simulink library "halout"  (R2021b)
settings: Solver=VariableStepAuto  StartTime=0.0  StopTime=10.0  RelTol=1e-3
undefined symbols (not defined in the file): C_TASK_5MS_S, FALSE, KHAL_CAN1TxReq_flg, KHAL_CAN2TxReq_flg, KHAL_CAN3FD3VCU1toNIDECTxReq_flg, KHAL_CAN3FD3VCU1TxReq_flg, KHAL_CAN3FD3VCU2E2E_flg, KHAL_CAN3FD3VCU2toNIDECE2E_flg, KHAL_CAN3FD3VCU2toNIDECTxReq_flg, KHAL_CAN3FD3VCU2TxReq_flg, KHAL_CAN3TxReq_flg, KHAL_CAN4FD4CE1000E2E_flg, KHAL_CAN4FD4CE1000TxReq_flg, KHAL_CAN4TxReq_flg, KHAL_CAN5TxReq_flg, KHAL_CAN7TxReq_flg, ONE_INT, TRUE, ZERO_INT
libraries: FVT_lib x258, simulink x115
(part 12 of 17)

== system halout/HAL_OUT/CAN3/FD3_THCM1_0x182/BatteryMode ==
  BatteryMode : Inport
  Data Type Conversion : DataTypeConversion  OutDataTypeStr=uint8  RndMeth=Round
  CAN3_BatteryMode : Outport
  wires:
  Data Type Conversion/1 -> CAN3_BatteryMode/1
  BatteryMode/1 -> Data Type Conversion/1

== system halout/HAL_OUT/CAN3/FD3_THCM1_0x182/CCUACLampSts ==
  CCUACLampSts : Inport
  Data Type Conversion : DataTypeConversion  OutDataTypeStr=uint8  RndMeth=Round
  CAN3_CCU_ACLampSts : Outport
  wires:
  Data Type Conversion/1 -> CAN3_CCU_ACLampSts/1
  CCUACLampSts/1 -> Data Type Conversion/1

== system halout/HAL_OUT/CAN3/FD3_THCM1_0x182/CCUACMaxLampSts ==
  CCUACMaxLampSts : Inport
  Data Type Conversion : DataTypeConversion  OutDataTypeStr=uint8  RndMeth=Round
  CAN3_CCU_ACMaxLampSts : Outport
  wires:
  Data Type Conversion/1 -> CAN3_CCU_ACMaxLampSts/1
  CCUACMaxLampSts/1 -> Data Type Conversion/1

== system halout/HAL_OUT/CAN3/FD3_THCM1_0x182/CCUAutoLampSts ==
  CCUAutoLampSts : Inport
  Data Type Conversion : DataTypeConversion  OutDataTypeStr=uint8  RndMeth=Round
  CAN3_CCU_AutoLampSts : Outport
  wires:
  Data Type Conversion/1 -> CAN3_CCU_AutoLampSts/1
  CCUAutoLampSts/1 -> Data Type Conversion/1

== system halout/HAL_OUT/CAN3/FD3_THCM1_0x182/CCUAutoMidLampSts ==
  CCUAutoMidLampSts : Inport
  Data Type Conversion : DataTypeConversion  OutDataTypeStr=uint8  RndMeth=Round
  CAN3_CCU_AutoMidLampSts : Outport
  wires:
  Data Type Conversion/1 -> CAN3_CCU_AutoMidLampSts/1
  CCUAutoMidLampSts/1 -> Data Type Conversion/1

== system halout/HAL_OUT/CAN3/FD3_THCM1_0x182/CCUDispalyRequest ==
  CCUDispalyRequest : Inport
  Data Type Conversion : DataTypeConversion  OutDataTypeStr=uint8  RndMeth=Round
  CAN3_CCU_Dispaly_Request : Outport
  wires:
  Data Type Conversion/1 -> CAN3_CCU_Dispaly_Request/1
  CCUDispalyRequest/1 -> Data Type Conversion/1

== system halout/HAL_OUT/CAN3/FD3_THCM1_0x182/CCUEcoSts ==
  CCUEcoSts : Inport
  Data Type Conversion : DataTypeConversion  OutDataTypeStr=uint8  RndMeth=Round
  CAN3_CCU_EcoSts : Outport
  wires:
  Data Type Conversion/1 -> CAN3_CCU_EcoSts/1
  CCUEcoSts/1 -> Data Type Conversion/1

== system halout/HAL_OUT/CAN3/FD3_THCM1_0x182/CCUFrtOnOffLampSts ==
  CCUFrtOnOffLampSts : Inport
  Data Type Conversion : DataTypeConversion  OutDataTypeStr=uint8  RndMeth=Round
  CAN3_CCU_FrtOnOffLampSts : Outport
  wires:
  Data Type Conversion/1 -> CAN3_CCU_FrtOnOffLampSts/1
  CCUFrtOnOffLampSts/1 -> Data Type Conversion/1

== system halout/HAL_OUT/CAN3/FD3_THCM1_0x182/CCUHEATMaxLampSts ==
  CCUHEATMaxLampSts : Inport
  Data Type Conversion : DataTypeConversion  OutDataTypeStr=uint8  RndMeth=Round
  CAN3_CCU_HEATMaxLampSts : Outport
  wires:
  Data Type Conversion/1 -> CAN3_CCU_HEATMaxLampSts/1
  CCUHEATMaxLampSts/1 -> Data Type Conversion/1

== system halout/HAL_OUT/CAN3/FD3_THCM1_0x182/CCURrOnOffLampSts ==
  CCURrOnOffLampSts : Inport
  Data Type Conversion : DataTypeConversion  OutDataTypeStr=uint8  RndMeth=Round
  CAN3_CCU_RrOnOffLampSts : Outport
  wires:
  Data Type Conversion/1 -> CAN3_CCU_RrOnOffLampSts/1
  CCURrOnOffLampSts/1 -> Data Type Conversion/1

== system halout/HAL_OUT/CAN3/FD3_THCM1_0x182/CCUSyncLampSts ==
  CCUSyncLampSts : Inport
  Data Type Conversion : DataTypeConversion  OutDataTypeStr=uint8  RndMeth=Round
  CAN3_CCU_SyncLampSts : Outport
  wires:
  Data Type Conversion/1 -> CAN3_CCU_SyncLampSts/1
  CCUSyncLampSts/1 -> Data Type Conversion/1

== system halout/HAL_OUT/CAN3/FD3_THCM1_0x182/CabinMode ==
  CabinMode : Inport
  Data Type Conversion : DataTypeConversion  OutDataTypeStr=uint8  RndMeth=Round
  CAN3_CabinMode : Outport
  wires:
  Data Type Conversion/1 -> CAN3_CabinMode/1
  CabinMode/1 -> Data Type Conversion/1

== system halout/HAL_OUT/CAN3/FD3_THCM1_0x182/EDriveMode ==
  EDriveMode : Inport
  Data Type Conversion : DataTypeConversion  OutDataTypeStr=uint8  RndMeth=Round
  CAN3_EDriveMode : Outport
  wires:
  Data Type Conversion/1 -> CAN3_EDriveMode/1
  EDriveMode/1 -> Data Type Conversion/1

== system halout/HAL_OUT/CAN3/FD3_THCM1_0x182/FDAGSCmd ==
  FDAGSCmd : Inport
  Data Type Conversion : DataTypeConversion  OutDataTypeStr=uint8  RndMeth=Round
  CAN3_FD_AGS_Cmd : Outport
  wires:
  Data Type Conversion/1 -> CAN3_FD_AGS_Cmd/1
  FDAGSCmd/1 -> Data Type Conversion/1

== system halout/HAL_OUT/CAN3/FD3_THCM1_0x182/FDRecyAutoCmd ==
  FDRecyAutoCmd : Inport
  Data Type Conversion : DataTypeConversion  OutDataTypeStr=uint8  RndMeth=Round
  CAN3_FD_RecyAuto_Cmd : Outport
  wires:
  Data Type Conversion/1 -> CAN3_FD_RecyAuto_Cmd/1
  FDRecyAutoCmd/1 -> Data Type Conversion/1

== system halout/HAL_OUT/CAN3/FD3_THCM1_0x182/FrCoolantflow ==
  FrCoolantflow : Inport
  Data Type Conversion : DataTypeConversion  OutDataTypeStr=uint8  RndMeth=Round
  convert_out : FVT_lib/hal/convert_out  gain=0.25  offset=0
  CAN3_Fr_Coolantflow : Outport
  wires:
  Data Type Conversion/1 -> CAN3_Fr_Coolantflow/1
  convert_out/1 -> Data Type Conversion/1
  FrCoolantflow/1 -> convert_out/1

== system halout/HAL_OUT/CAN3/FD3_THCM1_0x182/FrCoolanttemp ==
  FrCoolanttemp : Inport
  Data Type Conversion : DataTypeConversion  OutDataTypeStr=uint16  RndMeth=Round
  convert_out : FVT_lib/hal/convert_out  gain=1  offset=-40
  CAN3_Fr_Coolanttemp : Outport
  wires:
  Data Type Conversion/1 -> CAN3_Fr_Coolanttemp/1
  convert_out/1 -> Data Type Conversion/1
  FrCoolanttemp/1 -> convert_out/1

== system halout/HAL_OUT/CAN3/FD3_THCM1_0x182/HPThermalRecoveryReq ==
  HPThermalRecoveryReq : Inport
  Data Type Conversion : DataTypeConversion  OutDataTypeStr=uint8  RndMeth=Round
  CAN3_HPThermalRecoveryReq : Outport
  wires:
  Data Type Conversion/1 -> CAN3_HPThermalRecoveryReq/1
  HPThermalRecoveryReq/1 -> Data Type Conversion/1

== system halout/HAL_OUT/CAN3/FD3_THCM1_0x182/RrCoolantflow ==
  RrCoolantflow : Inport
  Data Type Conversion : DataTypeConversion  OutDataTypeStr=uint8  RndMeth=Round
  convert_out : FVT_lib/hal/convert_out  gain=0.25  offset=0
  CAN3_Rr_Coolantflow : Outport
  wires:
  Data Type Conversion/1 -> CAN3_Rr_Coolantflow/1
  convert_out/1 -> Data Type Conversion/1
  RrCoolantflow/1 -> convert_out/1

== system halout/HAL_OUT/CAN3/FD3_THCM1_0x182/RrCoolanttemp ==
  RrCoolanttemp : Inport
  Data Type Conversion : DataTypeConversion  OutDataTypeStr=uint16  RndMeth=Round
  convert_out : FVT_lib/hal/convert_out  gain=1  offset=-40
  CAN3_Rr_Coolanttemp : Outport
  wires:
  Data Type Conversion/1 -> CAN3_Rr_Coolanttemp/1
  convert_out/1 -> Data Type Conversion/1
  RrCoolanttemp/1 -> convert_out/1

== system halout/HAL_OUT/CAN3/FD3_THCM1_0x182/sigAirIntenZon1St ==
  sigAirIntenZon1St : Inport
  Data Type Conversion : DataTypeConversion  OutDataTypeStr=uint8  RndMeth=Round
  CAN3_sigAirIntenZon1St : Outport
  wires:
  Data Type Conversion/1 -> CAN3_sigAirIntenZon1St/1
  sigAirIntenZon1St/1 -> Data Type Conversion/1

== system halout/HAL_OUT/CAN3/FD3_THCM1_0x182/sigAirIntenZon3St ==
  sigAirIntenZon3St : Inport
  Data Type Conversion : DataTypeConversion  OutDataTypeStr=uint8  RndMeth=Round
  CAN3_sigAirIntenZon3St : Outport
  wires:
  Data Type Conversion/1 -> CAN3_sigAirIntenZon3St/1
  sigAirIntenZon3St/1 -> Data Type Conversion/1

== system halout/HAL_OUT/CAN3/FD3_THCM1_0x182/sigAmbAirT ==
  sigAmbAirT : Inport
  Data Type Conversion : DataTypeConversion  OutDataTypeStr=uint8  RndMeth=Round
  convert_out : FVT_lib/hal/convert_out  gain=0.5  offset=-40
  CAN3_sigAmbAirT : Outport
  wires:
  Data Type Conversion/1 -> CAN3_sigAmbAirT/1
  convert_out/1 -> Data Type Conversion/1
  sigAmbAirT/1 -> convert_out/1

== system halout/HAL_OUT/CAN3/FD3_THCM1_0x182/sigCbnAirT ==
  sigCbnAirT : Inport
  Data Type Conversion : DataTypeConversion  OutDataTypeStr=uint8  RndMeth=Round
  convert_out : FVT_lib/hal/convert_out  gain=0.5  offset=-40
  CAN3_sigCbnAirT : Outport
  wires:
  Data Type Conversion/1 -> CAN3_sigCbnAirT/1
  convert_out/1 -> Data Type Conversion/1
  sigCbnAirT/1 -> convert_out/1

== system halout/HAL_OUT/CAN3/FD3_THCM1_0x182/sigCbnPTCPwrAct ==
  sigCbnPTCPwrAct : Inport
  Data Type Conversion : DataTypeConversion  OutDataTypeStr=uint8  RndMeth=Round
  convert_out : FVT_lib/hal/convert_out  gain=50  offset=0
  CAN3_sigCbnPTCPwrAct : Outport
  wires:
  Data Type Conversion/1 -> CAN3_sigCbnPTCPwrAct/1
  convert_out/1 -> Data Type Conversion/1
  sigCbnPTCPwrAct/1 -> convert_out/1

== system halout/HAL_OUT/CAN3/FD3_THCM1_0x182/sigCbnSolarLeft ==
  sigCbnSolarLeft : Inport
  Data Type Conversion : DataTypeConversion  OutDataTypeStr=uint8  RndMeth=Round
  convert_out : FVT_lib/hal/convert_out  gain=5  offset=0
  CAN3_sigCbnSolarLeft : Outport
  wires:
  Data Type Conversion/1 -> CAN3_sigCbnSolarLeft/1
  convert_out/1 -> Data Type Conversion/1
  sigCbnSolarLeft/1 -> convert_out/1

== system halout/HAL_OUT/CAN3/FD3_THCM1_0x182/sigCbnSolarRight ==
  sigCbnSolarRight : Inport
  Data Type Conversion : DataTypeConversion  OutDataTypeStr=uint8  RndMeth=Round
  convert_out : FVT_lib/hal/convert_out  gain=5  offset=0
  CAN3_sigCbnSolarRight : Outport
  wires:
  Data Type Conversion/1 -> CAN3_sigCbnSolarRight/1
  convert_out/1 -> Data Type Conversion/1
  sigCbnSolarRight/1 -> convert_out/1

== system halout/HAL_OUT/CAN3/FD3_THCM1_0x182/sigClmtCmprPwrAct ==
  sigClmtCmprPwrAct : Inport
  Data Type Conversion : DataTypeConversion  OutDataTypeStr=uint8  RndMeth=Round
  convert_out : FVT_lib/hal/convert_out  gain=50  offset=0
  CAN3_sigClmtCmprPwrAct : Outport
  wires:
  Data Type Conversion/1 -> CAN3_sigClmtCmprPwrAct/1
  convert_out/1 -> Data Type Conversion/1
  sigClmtCmprPwrAct/1 -> convert_out/1

== system halout/HAL_OUT/CAN3/FD3_THCM1_0x182/sigClntTHvBattOut ==
  sigClntTHvBattOut : Inport
  Data Type Conversion : DataTypeConversion  OutDataTypeStr=uint8  RndMeth=Round
  convert_out : FVT_lib/hal/convert_out  gain=0.5  offset=-40
  CAN3_sigClntTHvBattOut : Outport
  wires:
  Data Type Conversion/1 -> CAN3_sigClntTHvBattOut/1
  convert_out/1 -> Data Type Conversion/1
  sigClntTHvBattOut/1 -> convert_out/1

== system halout/HAL_OUT/CAN3/FD3_THCM1_0x182/sigDfrstSt ==
  sigDfrstSt : Inport
  Data Type Conversion : DataTypeConversion  OutDataTypeStr=uint8  RndMeth=Round
  CAN3_sigDfrstSt : Outport
  wires:
  Data Type Conversion/1 -> CAN3_sigDfrstSt/1
  sigDfrstSt/1 -> Data Type Conversion/1

== system halout/HAL_OUT/CAN3/FD3_THCM1_0x182/sigHvacSt ==
  sigHvacSt : Inport
  Data Type Conversion : DataTypeConversion  OutDataTypeStr=uint8  RndMeth=Round
  CAN3_sigHvacSt : Outport
  wires:
  Data Type Conversion/1 -> CAN3_sigHvacSt/1
  sigHvacSt/1 -> Data Type Conversion/1

== system halout/HAL_OUT/CAN3/FD3_THCM1_0x182/sigRecircSt ==
  sigRecircSt : Inport
  Data Type Conversion : DataTypeConversion  OutDataTypeStr=uint8  RndMeth=Round
  CAN3_sigRecircSt : Outport
  wires:
  Data Type Conversion/1 -> CAN3_sigRecircSt/1
  sigRecircSt/1 -> Data Type Conversion/1

== system halout/HAL_OUT/CAN3/FD3_THCM1_0x182/sigSetTempZon1St ==
  sigSetTempZon1St : Inport
  Data Type Conversion : DataTypeConversion  OutDataTypeStr=uint8  RndMeth=Round
  convert_out : FVT_lib/hal/convert_out  gain=0.5  offset=17
  CAN3_sigSetTempZon1St : Outport
  wires:
  Data Type Conversion/1 -> CAN3_sigSetTempZon1St/1
  convert_out/1 -> Data Type Conversion/1
  sigSetTempZon1St/1 -> convert_out/1

== system halout/HAL_OUT/CAN3/FD3_THCM1_0x182/sigSetTempZon2St ==
  sigSetTempZon2St : Inport
  Data Type Conversion : DataTypeConversion  OutDataTypeStr=uint8  RndMeth=Round
  convert_out : FVT_lib/hal/convert_out  gain=0.5  offset=17
  CAN3_sigSetTempZon2St : Outport
  wires:
  Data Type Conversion/1 -> CAN3_sigSetTempZon2St/1
  convert_out/1 -> Data Type Conversion/1
  sigSetTempZon2St/1 -> convert_out/1

== system halout/HAL_OUT/CAN3/FD3_THCM1_0x182/sigSetTempZon3St ==
  sigSetTempZon3St : Inport
  Data Type Conversion : DataTypeConversion  OutDataTypeStr=uint8  RndMeth=Round
  convert_out : FVT_lib/hal/convert_out  gain=0.5  offset=17
  CAN3_sigSetTempZon3St : Outport
  wires:
  Data Type Conversion/1 -> CAN3_sigSetTempZon3St/1
  convert_out/1 -> Data Type Conversion/1
  sigSetTempZon3St/1 -> convert_out/1

== system halout/HAL_OUT/CAN3/FD3_THCM1_0x182/sigWindDirZon1St ==
  sigWindDirZon1St : Inport
  Data Type Conversion : DataTypeConversion  OutDataTypeStr=uint8  RndMeth=Round
  CAN3_sigWindDirZon1St : Outport
  wires:
  Data Type Conversion/1 -> CAN3_sigWindDirZon1St/1
  sigWindDirZon1St/1 -> Data Type Conversion/1

== system halout/HAL_OUT/CAN3/FD3_THCM1_0x182/sigWindDirZon3St ==
  sigWindDirZon3St : Inport
  Data Type Conversion : DataTypeConversion  OutDataTypeStr=uint8  RndMeth=Round
  CAN3_sigWindDirZon3St : Outport
  wires:
  Data Type Conversion/1 -> CAN3_sigWindDirZon3St/1
  sigWindDirZon3St/1 -> Data Type Conversion/1

== system halout/HAL_OUT/CAN3/FD3_THCM2_0x186/ACSubMode ==
  ACSubMode : Inport
  Data Type Conversion : DataTypeConversion  OutDataTypeStr=uint8  RndMeth=Round
  CAN3_ACSubMode : Outport
  wires:
  Data Type Conversion/1 -> CAN3_ACSubMode/1
  ACSubMode/1 -> Data Type Conversion/1

== system halout/HAL_OUT/CAN3/FD3_THCM2_0x186/APTCActFrRiPwr ==
  APTCActFrRiPwr : Inport
  Data Type Conversion : DataTypeConversion  OutDataTypeStr=uint8  RndMeth=Round
  convert_out : FVT_lib/hal/convert_out  gain=25  offset=0
  CAN3_APTC_ActFrRiPwr : Outport
  wires:
  Data Type Conversion/1 -> CAN3_APTC_ActFrRiPwr/1
  convert_out/1 -> Data Type Conversion/1
  APTCActFrRiPwr/1 -> convert_out/1

== system halout/HAL_OUT/CAN3/FD3_THCM2_0x186/BatLoopActWtFlw ==
  BatLoopActWtFlw : Inport
  Data Type Conversion : DataTypeConversion  OutDataTypeStr=uint8  RndMeth=Round
  convert_out : FVT_lib/hal/convert_out  gain=0.1  offset=-5
  CAN3_BatLoopActWtFlw : Outport
  wires:
  Data Type Conversion/1 -> CAN3_BatLoopActWtFlw/1
  convert_out/1 -> Data Type Conversion/1
  BatLoopActWtFlw/1 -> convert_out/1

== system halout/HAL_OUT/CAN3/FD3_THCM2_0x186/CCUCbnPreACWkSts ==
  CCUCbnPreACWkSts : Inport
  Data Type Conversion : DataTypeConversion  OutDataTypeStr=uint8  RndMeth=Round
  CAN3_CCU_CbnPreACWkSts : Outport
  wires:
  Data Type Conversion/1 -> CAN3_CCU_CbnPreACWkSts/1
  CCUCbnPreACWkSts/1 -> Data Type Conversion/1

== system halout/HAL_OUT/CAN3/FD3_THCM2_0x186/CCUCbnPreEstimdTi ==
  CCUCbnPreEstimdTi : Inport
  Data Type Conversion : DataTypeConversion  OutDataTypeStr=uint8  RndMeth=Round
  CAN3_CCU_CbnPreEstimdTi : Outport
  wires:
  Data Type Conversion/1 -> CAN3_CCU_CbnPreEstimdTi/1
  CCUCbnPreEstimdTi/1 -> Data Type Conversion/1

== system halout/HAL_OUT/CAN3/FD3_THCM2_0x186/CCUCbnPreSts ==
  CCUCbnPreSts : Inport
  Data Type Conversion : DataTypeConversion  OutDataTypeStr=uint8  RndMeth=Round
  CAN3_CCU_CbnPreSts : Outport
  wires:
  Data Type Conversion/1 -> CAN3_CCU_CbnPreSts/1
  CCUCbnPreSts/1 -> Data Type Conversion/1

== system halout/HAL_OUT/CAN3/FD3_THCM2_0x186/CCUHiVoltageReq ==
  CCUHiVoltageReq : Inport
  Data Type Conversion : DataTypeConversion  OutDataTypeStr=uint8  RndMeth=Round
  CAN3_CCU_HiVoltageReq : Outport
  wires:
  Data Type Conversion/1 -> CAN3_CCU_HiVoltageReq/1
  CCUHiVoltageReq/1 -> Data Type Conversion/1

== system halout/HAL_OUT/CAN3/FD3_THCM2_0x186/CoolgFanActDuty ==
  CoolgFanActDuty : Inport
  Data Type Conversion : DataTypeConversion  OutDataTypeStr=uint8  RndMeth=Round
  convert_out : FVT_lib/hal/convert_out  gain=0.5  offset=0
  CAN3_CoolgFanActDuty : Outport
  wires:
  Data Type Conversion/1 -> CAN3_CoolgFanActDuty/1
  convert_out/1 -> Data Type Conversion/1
  CoolgFanActDuty/1 -> convert_out/1

== system halout/HAL_OUT/CAN3/FD3_THCM2_0x186/DeiceModReq ==
  DeiceModReq : Inport
  Data Type Conversion : DataTypeConversion  OutDataTypeStr=uint8  RndMeth=Round
  CAN3_DeiceModReq : Outport
  wires:
  Data Type Conversion/1 -> CAN3_DeiceModReq/1
  DeiceModReq/1 -> Data Type Conversion/1

== system halout/HAL_OUT/CAN3/FD3_THCM2_0x186/FDBlowerCmd ==
  FDBlowerCmd : Inport
  Data Type Conversion : DataTypeConversion  OutDataTypeStr=uint8  RndMeth=Round
  convert_out : FVT_lib/hal/convert_out  gain=0.8  offset=0
  CAN3_FD_Blower_Cmd : Outport
  wires:
  Data Type Conversion/1 -> CAN3_FD_Blower_Cmd/1
  convert_out/1 -> Data Type Conversion/1
  FDBlowerCmd/1 -> convert_out/1

== system halout/HAL_OUT/CAN3/FD3_THCM2_0x186/FDCompCmd ==
  FDCompCmd : Inport
  Data Type Conversion : DataTypeConversion  OutDataTypeStr=uint16  RndMeth=Round
  convert_out : FVT_lib/hal/convert_out  gain=0.5  offset=0
  CAN3_FD_Comp_Cmd : Outport
  wires:
  Data Type Conversion/1 -> CAN3_FD_Comp_Cmd/1
  convert_out/1 -> Data Type Conversion/1
  FDCompCmd/1 -> convert_out/1

== system halout/HAL_OUT/CAN3/FD3_THCM2_0x186/FDEWP1Cmd ==
  FDEWP1Cmd : Inport
  Data Type Conversion : DataTypeConversion  OutDataTypeStr=uint8  RndMeth=Round
  CAN3_FD_EWP1_Cmd : Outport
  wires:
  Data Type Conversion/1 -> CAN3_FD_EWP1_Cmd/1
  FDEWP1Cmd/1 -> Data Type Conversion/1

== system halout/HAL_OUT/CAN3/FD3_THCM2_0x186/FDEWP2Cmd ==
  FDEWP2Cmd : Inport
  Data Type Conversion : DataTypeConversion  OutDataTypeStr=uint8  RndMeth=Round
  CAN3_FD_EWP2_Cmd : Outport
  wires:
  Data Type Conversion/1 -> CAN3_FD_EWP2_Cmd/1
  FDEWP2Cmd/1 -> Data Type Conversion/1

== system halout/HAL_OUT/CAN3/FD3_THCM2_0x186/FDEWP3Cmd ==
  FDEWP3Cmd : Inport
  Data Type Conversion : DataTypeConversion  OutDataTypeStr=uint8  RndMeth=Round
  CAN3_FD_EWP3_Cmd : Outport
  wires:
  Data Type Conversion/1 -> CAN3_FD_EWP3_Cmd/1
  FDEWP3Cmd/1 -> Data Type Conversion/1

== system halout/HAL_OUT/CAN3/FD3_THCM2_0x186/FDEXV1Cmd ==
  FDEXV1Cmd : Inport
  Data Type Conversion : DataTypeConversion  OutDataTypeStr=uint16  RndMeth=Round
  CAN3_FD_EXV1_Cmd : Outport
  wires:
  Data Type Conversion/1 -> CAN3_FD_EXV1_Cmd/1
  FDEXV1Cmd/1 -> Data Type Conversion/1

== system halout/HAL_OUT/CAN3/FD3_THCM2_0x186/FDEXV2Cmd ==
  FDEXV2Cmd : Inport
  Data Type Conversion : DataTypeConversion  OutDataTypeStr=uint16  RndMeth=Round
  CAN3_FD_EXV2_Cmd : Outport
  wires:
  Data Type Conversion/1 -> CAN3_FD_EXV2_Cmd/1
  FDEXV2Cmd/1 -> Data Type Conversion/1

== system halout/HAL_OUT/CAN3/FD3_THCM2_0x186/FDFWVCmd ==
  FDFWVCmd : Inport
  Data Type Conversion : DataTypeConversion  OutDataTypeStr=uint8  RndMeth=Round
  CAN3_FD_FWV_Cmd : Outport
  wires:
  Data Type Conversion/1 -> CAN3_FD_FWV_Cmd/1
  FDFWVCmd/1 -> Data Type Conversion/1

== system halout/HAL_OUT/CAN3/FD3_THCM2_0x186/FDFrLeAPTCHeatPwrCmd ==
  FDFrLeAPTCHeatPwrCmd : Inport
  Data Type Conversion : DataTypeConversion  OutDataTypeStr=uint8  RndMeth=Round
  convert_out : FVT_lib/hal/convert_out  gain=25  offset=0
  CAN3_FD_FrLeAPTCHeatPwr_Cmd : Outport
  wires:
  Data Type Conversion/1 -> CAN3_FD_FrLeAPTCHeatPwr_Cmd/1
  convert_out/1 -> Data Type Conversion/1
  FDFrLeAPTCHeatPwrCmd/1 -> convert_out/1

== system halout/HAL_OUT/CAN3/FD3_THCM2_0x186/FDFrRiAPTCHeatPwrCmd ==
  FDFrRiAPTCHeatPwrCmd : Inport
  Data Type Conversion : DataTypeConversion  OutDataTypeStr=uint8  RndMeth=Round
  convert_out : FVT_lib/hal/convert_out  gain=25  offset=0
  CAN3_FD_FrRiAPTCHeatPwr_Cmd : Outport
  wires:
  Data Type Conversion/1 -> CAN3_FD_FrRiAPTCHeatPwr_Cmd/1
  convert_out/1 -> Data Type Conversion/1
  FDFrRiAPTCHeatPwrCmd/1 -> convert_out/1

== system halout/HAL_OUT/CAN3/FD3_THCM2_0x186/FDFrWPTCHeatPwrCmd ==
  FDFrWPTCHeatPwrCmd : Inport
  Data Type Conversion : DataTypeConversion  OutDataTypeStr=uint16  RndMeth=Round
  CAN3_FD_FrWPTCHeatPwr_Cmd : Outport
  wires:
  Data Type Conversion/1 -> CAN3_FD_FrWPTCHeatPwr_Cmd/1
  FDFrWPTCHeatPwrCmd/1 -> Data Type Conversion/1

== system halout/HAL_OUT/CAN3/FD3_THCM2_0x186/FDRrAPTCHeatPwrCmd ==
  FDRrAPTCHeatPwrCmd : Inport
  Data Type Conversion : DataTypeConversion  OutDataTypeStr=uint8  RndMeth=Round
  convert_out : FVT_lib/hal/convert_out  gain=25  offset=0
  CAN3_FD_RrAPTCHeatPwr_Cmd : Outport
  wires:
  Data Type Conversion/1 -> CAN3_FD_RrAPTCHeatPwr_Cmd/1
  convert_out/1 -> Data Type Conversion/1
  FDRrAPTCHeatPwrCmd/1 -> convert_out/1

== system halout/HAL_OUT/CAN3/FD3_THCM2_0x186/FDSOTXVCmd ==
  FDSOTXVCmd : Inport
  Data Type Conversion : DataTypeConversion  OutDataTypeStr=uint8  RndMeth=Round
  CAN3_FD_SOTXV_Cmd : Outport
  wires:
  Data Type Conversion/1 -> CAN3_FD_SOTXV_Cmd/1
  FDSOTXVCmd/1 -> Data Type Conversion/1

== system halout/HAL_OUT/CAN3/FD3_THCM2_0x186/FDSOV1Cmd ==
  FDSOV1Cmd : Inport
  Data Type Conversion : DataTypeConversion  OutDataTypeStr=uint8  RndMeth=Round
  CAN3_FD_SOV1_Cmd : Outport
  wires:
  Data Type Conversion/1 -> CAN3_FD_SOV1_Cmd/1
  FDSOV1Cmd/1 -> Data Type Conversion/1

== system halout/HAL_OUT/CAN3/FD3_THCM2_0x186/FDSOV2Cmd ==
  FDSOV2Cmd : Inport
  Data Type Conversion : DataTypeConversion  OutDataTypeStr=uint8  RndMeth=Round
  CAN3_FD_SOV2_Cmd : Outport
  wires:
  Data Type Conversion/1 -> CAN3_FD_SOV2_Cmd/1
  FDSOV2Cmd/1 -> Data Type Conversion/1

== system halout/HAL_OUT/CAN3/FD3_THCM2_0x186/FDSOV3Cmd ==
  FDSOV3Cmd : Inport
  Data Type Conversion : DataTypeConversion  OutDataTypeStr=uint8  RndMeth=Round
  CAN3_FD_SOV3_Cmd : Outport
  wires:
  Data Type Conversion/1 -> CAN3_FD_SOV3_Cmd/1
  FDSOV3Cmd/1 -> Data Type Conversion/1

== system halout/HAL_OUT/CAN3/FD3_THCM2_0x186/FDTWVCmd ==
  FDTWVCmd : Inport
  Data Type Conversion : DataTypeConversion  OutDataTypeStr=uint8  RndMeth=Round
  convert_out : FVT_lib/hal/convert_out  gain=0.392  offset=0
  CAN3_FD_TWV_Cmd : Outport
  wires:
  Data Type Conversion/1 -> CAN3_FD_TWV_Cmd/1
  convert_out/1 -> Data Type Conversion/1
  FDTWVCmd/1 -> convert_out/1

== system halout/HAL_OUT/CAN3/FD3_V2L1_0x374/ReqOBCV2LEna ==
  ReqOBCV2LEna : Inport
  Data Type Conversion : DataTypeConversion  OutDataTypeStr=uint8  RndMeth=Round
  CAN3_Req_OBCV2LEna : Outport
  wires:
  Data Type Conversion/1 -> CAN3_Req_OBCV2LEna/1
  ReqOBCV2LEna/1 -> Data Type Conversion/1

== system halout/HAL_OUT/CAN3/FD3_V2L1_0x374/ReqV2LIVIPopup ==
  ReqV2LIVIPopup : Inport
  Data Type Conversion : DataTypeConversion  OutDataTypeStr=uint8  RndMeth=Round
  CAN3_Req_V2L_IVI_Popup : Outport
  wires:
  Data Type Conversion/1 -> CAN3_Req_V2L_IVI_Popup/1
  ReqV2LIVIPopup/1 -> Data Type Conversion/1

== system halout/HAL_OUT/CAN3/FD3_V2L1_0x374/ReqV2LSwOn ==
  ReqV2LSwOn : Inport
  Data Type Conversion : DataTypeConversion  OutDataTypeStr=uint8  RndMeth=Round
  CAN3_Req_V2LSwOn : Outport
  wires:
  Data Type Conversion/1 -> CAN3_Req_V2LSwOn/1
  ReqV2LSwOn/1 -> Data Type Conversion/1

== system halout/HAL_OUT/CAN3/FD3_VCU0_0x1F0/EVCCAplusPwrUpReq ==
  EVCCAplusPwrUpReq : Inport
  Data Type Conversion : DataTypeConversion  OutDataTypeStr=uint8  RndMeth=Round
  CAN3_EVCCAplusPwrUpReq : Outport
  wires:
  Data Type Conversion/1 -> CAN3_EVCCAplusPwrUpReq/1
  EVCCAplusPwrUpReq/1 -> Data Type Conversion/1

== system halout/HAL_OUT/CAN3/FD3_VCU0_0x1F0/FDADC12VDet ==
  FDADC12VDet : Inport
  Data Type Conversion : DataTypeConversion  OutDataTypeStr=uint8  RndMeth=Round
  convert_out : FVT_lib/hal/convert_out  gain=0.1  offset=0
  CAN3_FDADC12VDet : Outport
  wires:
  Data Type Conversion/1 -> CAN3_FDADC12VDet/1
  convert_out/1 -> Data Type Conversion/1
  FDADC12VDet/1 -> convert_out/1

== system halout/HAL_OUT/CAN3/FD3_VCU0_0x1F0/FDADC12VDetAvg ==
  FDADC12VDetAvg : Inport
  Data Type Conversion : DataTypeConversion  OutDataTypeStr=uint8  RndMeth=Round
  convert_out : FVT_lib/hal/convert_out  gain=0.1  offset=0
  CAN3_FDADC12VDetAvg : Outport
  wires:
  Data Type Conversion/1 -> CAN3_FDADC12VDetAvg/1
  convert_out/1 -> Data Type Conversion/1
  FDADC12VDetAvg/1 -> convert_out/1

== system halout/HAL_OUT/CAN3/FD3_VCU0_0x1F0/FDCVCUActMaxSlideRateSta ==
  FDCVCUActMaxSlideRateSta : Inport
  Data Type Conversion : DataTypeConversion  OutDataTypeStr=uint16  RndMeth=Round
  convert_out : FVT_lib/hal/convert_out  gain=0.01  offset=-150
  CAN3_FDC_VCU_ActMaxSlideRate_Sta : Outport
  wires:
  Data Type Conversion/1 -> CAN3_FDC_VCU_ActMaxSlideRate_Sta/1
  convert_out/1 -> Data Type Conversion/1
  FDCVCUActMaxSlideRateSta/1 -> convert_out/1

== system halout/HAL_OUT/CAN3/FD3_VCU0_0x1F0/FDCVCUAllowMovThdOTASta ==
  FDCVCUAllowMovThdOTASta : Inport
  Data Type Conversion : DataTypeConversion  OutDataTypeStr=uint8  RndMeth=Round
  CAN3_FDC_VCU_AllowMovThd_OTA_Sta : Outport
  wires:
  Data Type Conversion/1 -> CAN3_FDC_VCU_AllowMovThd_OTA_Sta/1
  FDCVCUAllowMovThdOTASta/1 -> Data Type Conversion/1

== system halout/HAL_OUT/CAN3/FD3_VCU0_0x1F0/FDCVCUDTCCarouselSta ==
  FDCVCUDTCCarouselSta : Inport
  Data Type Conversion : DataTypeConversion  OutDataTypeStr=uint8  RndMeth=Round
  CAN3_FDC_VCU_DTCCarousel_Sta : Outport
  wires:
  Data Type Conversion/1 -> CAN3_FDC_VCU_DTCCarousel_Sta/1
  FDCVCUDTCCarouselSta/1 -> Data Type Conversion/1

== system halout/HAL_OUT/CAN3/FD3_VCU0_0x1F0/FDCVCUForcePCmd ==
  FDCVCUForcePCmd : Inport
  Data Type Conversion : DataTypeConversion  OutDataTypeStr=uint8  RndMeth=Round
  CAN3_FDC_VCU_ForceP_Cmd : Outport
  wires:
  Data Type Conversion/1 -> CAN3_FDC_VCU_ForceP_Cmd/1
  FDCVCUForcePCmd/1 -> Data Type Conversion/1

== system halout/HAL_OUT/CAN3/FD3_VCU0_0x1F0/FDCVCUOTAPwrReqOFFChkSta ==
  FDCVCUOTAPwrReqOFFChkSta : Inport
  Data Type Conversion : DataTypeConversion  OutDataTypeStr=uint8  RndMeth=Round
  CAN3_FDC_VCU_OTAPwrReqOFFChk_Sta : Outport
  wires:
  Data Type Conversion/1 -> CAN3_FDC_VCU_OTAPwrReqOFFChk_Sta/1
  FDCVCUOTAPwrReqOFFChkSta/1 -> Data Type Conversion/1

== system halout/HAL_OUT/CAN3/FD3_VCU0_0x1F0/FDCVCUOTAPwrReqStdChkSta ==
  FDCVCUOTAPwrReqStdChkSta : Inport
  Data Type Conversion : DataTypeConversion  OutDataTypeStr=uint8  RndMeth=Round
  CAN3_FDC_VCU_OTAPwrReqStdChk_Sta : Outport
  wires:
  Data Type Conversion/1 -> CAN3_FDC_VCU_OTAPwrReqStdChk_Sta/1
  FDCVCUOTAPwrReqStdChkSta/1 -> Data Type Conversion/1

== system halout/HAL_OUT/CAN3/FD3_VCU0_0x1F0/FDCVCUPwrReqOTASta ==
  FDCVCUPwrReqOTASta : Inport
  Data Type Conversion : DataTypeConversion  OutDataTypeStr=uint8  RndMeth=Round
  CAN3_FDC_VCU_PwrReq_OTA_Sta : Outport
  wires:
  Data Type Conversion/1 -> CAN3_FDC_VCU_PwrReq_OTA_Sta/1
  FDCVCUPwrReqOTASta/1 -> Data Type Conversion/1

== system halout/HAL_OUT/CAN3/FD3_VCU0_0x1F0/FDCVCURWDRDCActiveSta ==
  FDCVCURWDRDCActiveSta : Inport
  Data Type Conversion : DataTypeConversion  OutDataTypeStr=uint8  RndMeth=Round
  CAN3_FDC_VCU_RWDRDCActive_Sta : Outport
  wires:
  Data Type Conversion/1 -> CAN3_FDC_VCU_RWDRDCActive_Sta/1
  FDCVCURWDRDCActiveSta/1 -> Data Type Conversion/1

== system halout/HAL_OUT/CAN3/FD3_VCU0_0x1F0/FDCVCURegenTqLimitEnSta ==
  FDCVCURegenTqLimitEnSta : Inport
  Data Type Conversion : DataTypeConversion  OutDataTypeStr=uint8  RndMeth=Round
  CAN3_FDC_VCU_RegenTqLimitEn_Sta : Outport
  wires:
  Data Type Conversion/1 -> CAN3_FDC_VCU_RegenTqLimitEn_Sta/1
  FDCVCURegenTqLimitEnSta/1 -> Data Type Conversion/1

== system halout/HAL_OUT/CAN3/FD3_VCU0_0x1F0/FDCVCUSlideRegenLimTqSta ==
  FDCVCUSlideRegenLimTqSta : Inport
  Data Type Conversion : DataTypeConversion  OutDataTypeStr=uint16  RndMeth=Round
  convert_out : FVT_lib/hal/convert_out  gain=0.5  offset=-5300
  CAN3_FDC_VCU_SlideRegenLimTq_Sta : Outport
  wires:
  Data Type Conversion/1 -> CAN3_FDC_VCU_SlideRegenLimTq_Sta/1
  convert_out/1 -> Data Type Conversion/1
  FDCVCUSlideRegenLimTqSta/1 -> convert_out/1

== system halout/HAL_OUT/CAN3/FD3_VCU0_0x1F0/FDCVCUVehActSpdSta ==
  FDCVCUVehActSpdSta : Inport
  Data Type Conversion : DataTypeConversion  OutDataTypeStr=uint16  RndMeth=Round
  convert_out : FVT_lib/hal/convert_out  gain=0.01  offset=-300
  CAN3_FDC_VCU_VehActSpd_Sta : Outport
  wires:
  Data Type Conversion/1 -> CAN3_FDC_VCU_VehActSpd_Sta/1
  convert_out/1 -> Data Type Conversion/1
  FDCVCUVehActSpdSta/1 -> convert_out/1

== system halout/HAL_OUT/CAN3/FD3_VCU0_0x1F0/FDCVCUVehMalfunLevelSta ==
  FDCVCUVehMalfunLevelSta : Inport
  Data Type Conversion : DataTypeConversion  OutDataTypeStr=uint8  RndMeth=Round
  CAN3_FDC_VCU_VehMalfunLevel_Sta : Outport
  wires:
  Data Type Conversion/1 -> CAN3_FDC_VCU_VehMalfunLevel_Sta/1
  FDCVCUVehMalfunLevelSta/1 -> Data Type Conversion/1

== system halout/HAL_OUT/CAN3/FD3_VCU0_0x1F0/FDCVMCActStESCYawSta ==
  FDCVMCActStESCYawSta : Inport
  Data Type Conversion : DataTypeConversion  OutDataTypeStr=uint16  RndMeth=Round
  convert_out : FVT_lib/hal/convert_out  gain=0.01  offset=-300
  CAN3_FDC_VMC_ActStESCYaw_Sta : Outport
  wires:
  Data Type Conversion/1 -> CAN3_FDC_VMC_ActStESCYaw_Sta/1
  convert_out/1 -> Data Type Conversion/1
  FDCVMCActStESCYawSta/1 -> convert_out/1

== system halout/HAL_OUT/CAN3/FD3_VCU0_0x1F0/FDCVMCLongAccSta ==
  FDCVMCLongAccSta : Inport
  Data Type Conversion : DataTypeConversion  OutDataTypeStr=uint16  RndMeth=Round
  convert_out : FVT_lib/hal/convert_out  gain=0.001  offset=-20
  CAN3_FDC_VMC_LongAcc_Sta : Outport
  wires:
  Data Type Conversion/1 -> CAN3_FDC_VMC_LongAcc_Sta/1
  convert_out/1 -> Data Type Conversion/1
  FDCVMCLongAccSta/1 -> convert_out/1

== system halout/HAL_OUT/CAN3/FD3_VCU0_0x1F0/FUSIONCMM1 ==
  FUSIONCMM1 : Inport
  Data Type Conversion : DataTypeConversion  OutDataTypeStr=uint8  RndMeth=Round
  CAN3_FUSION_CMM1 : Outport
  wires:
  Data Type Conversion/1 -> CAN3_FUSION_CMM1/1
  FUSIONCMM1/1 -> Data Type Conversion/1

== system halout/HAL_OUT/CAN3/FD3_VCU0_0x1F0/FUSIONCMM10 ==
  FUSIONCMM10 : Inport
  Data Type Conversion : DataTypeConversion  OutDataTypeStr=uint8  RndMeth=Round
  CAN3_FUSION_CMM10 : Outport
  wires:
  Data Type Conversion/1 -> CAN3_FUSION_CMM10/1
  FUSIONCMM10/1 -> Data Type Conversion/1

== system halout/HAL_OUT/CAN3/FD3_VCU0_0x1F0/FUSIONCMM2 ==
  FUSIONCMM2 : Inport
  Data Type Conversion : DataTypeConversion  OutDataTypeStr=uint8  RndMeth=Round
  CAN3_FUSION_CMM2 : Outport
  wires:
  Data Type Conversion/1 -> CAN3_FUSION_CMM2/1
  FUSIONCMM2/1 -> Data Type Conversion/1

== system halout/HAL_OUT/CAN3/FD3_VCU0_0x1F0/FUSIONCMM3 ==
  FUSIONCMM3 : Inport
  Data Type Conversion : DataTypeConversion  OutDataTypeStr=uint8  RndMeth=Round
  CAN3_FUSION_CMM3 : Outport
  wires:
  Data Type Conversion/1 -> CAN3_FUSION_CMM3/1
  FUSIONCMM3/1 -> Data Type Conversion/1

== system halout/HAL_OUT/CAN3/FD3_VCU0_0x1F0/FUSIONCMM4 ==
  FUSIONCMM4 : Inport
  Data Type Conversion : DataTypeConversion  OutDataTypeStr=uint8  RndMeth=Round
  CAN3_FUSION_CMM4 : Outport
  wires:
  Data Type Conversion/1 -> CAN3_FUSION_CMM4/1
  FUSIONCMM4/1 -> Data Type Conversion/1

== system halout/HAL_OUT/CAN3/FD3_VCU0_0x1F0/FUSIONCMM5 ==
  FUSIONCMM5 : Inport
  Data Type Conversion : DataTypeConversion  OutDataTypeStr=uint8  RndMeth=Round
  CAN3_FUSION_CMM5 : Outport
  wires:
  Data Type Conversion/1 -> CAN3_FUSION_CMM5/1
  FUSIONCMM5/1 -> Data Type Conversion/1

== system halout/HAL_OUT/CAN3/FD3_VCU0_0x1F0/FUSIONCMM6 ==
  FUSIONCMM6 : Inport
  Data Type Conversion : DataTypeConversion  OutDataTypeStr=uint8  RndMeth=Round
  CAN3_FUSION_CMM6 : Outport
  wires:
  Data Type Conversion/1 -> CAN3_FUSION_CMM6/1
  FUSIONCMM6/1 -> Data Type Conversion/1

== system halout/HAL_OUT/CAN3/FD3_VCU0_0x1F0/FUSIONCMM7 ==
  FUSIONCMM7 : Inport
  Data Type Conversion : DataTypeConversion  OutDataTypeStr=uint8  RndMeth=Round
  CAN3_FUSION_CMM7 : Outport
  wires:
  Data Type Conversion/1 -> CAN3_FUSION_CMM7/1
  FUSIONCMM7/1 -> Data Type Conversion/1

== system halout/HAL_OUT/CAN3/FD3_VCU0_0x1F0/FUSIONCMM8 ==
  FUSIONCMM8 : Inport
  Data Type Conversion : DataTypeConversion  OutDataTypeStr=uint8  RndMeth=Round
  CAN3_FUSION_CMM8 : Outport
  wires:
  Data Type Conversion/1 -> CAN3_FUSION_CMM8/1
  FUSIONCMM8/1 -> Data Type Conversion/1

== system halout/HAL_OUT/CAN3/FD3_VCU0_0x1F0/FUSIONCMM9 ==
  FUSIONCMM9 : Inport
  Data Type Conversion : DataTypeConversion  OutDataTypeStr=uint8  RndMeth=Round
  CAN3_FUSION_CMM9 : Outport
  wires:
  Data Type Conversion/1 -> CAN3_FUSION_CMM9/1
  FUSIONCMM9/1 -> Data Type Conversion/1

== system halout/HAL_OUT/CAN3/FD3_VCU0_0x1F0/FrTqSource ==
  FrTqSource : Inport
  Data Type Conversion : DataTypeConversion  OutDataTypeStr=uint8  RndMeth=Round
  CAN3_Fr_TqSource : Outport
  wires:
  Data Type Conversion/1 -> CAN3_Fr_TqSource/1
  FrTqSource/1 -> Data Type Conversion/1

== system halout/HAL_OUT/CAN3/FD3_VCU0_0x1F0/HVRlyOpFail ==
  HVRlyOpFail : Inport
  Data Type Conversion : DataTypeConversion  OutDataTypeStr=uint8  RndMeth=Round
  CAN3_HVRlyOpFail : Outport
  wires:
  Data Type Conversion/1 -> CAN3_HVRlyOpFail/1
  HVRlyOpFail/1 -> Data Type Conversion/1

== system halout/HAL_OUT/CAN3/FD3_VCU0_0x1F0/HVTHCMSysAvail ==
  HVTHCMSysAvail : Inport
  Data Type Conversion : DataTypeConversion  OutDataTypeStr=uint8  RndMeth=Round
  CAN3_HVTHCMSysAvail : Outport
  wires:
  Data Type Conversion/1 -> CAN3_HVTHCMSysAvail/1
  HVTHCMSysAvail/1 -> Data Type Conversion/1

== system halout/HAL_OUT/CAN3/FD3_VCU0_0x1F0/LVBattChrgtimeAct ==
  LVBattChrgtimeAct : Inport
  Data Type Conversion : DataTypeConversion  OutDataTypeStr=uint16  RndMeth=Round
  CAN3_LVBattChrgtimeAct : Outport
  wires:
  Data Type Conversion/1 -> CAN3_LVBattChrgtimeAct/1
  LVBattChrgtimeAct/1 -> Data Type Conversion/1

== system halout/HAL_OUT/CAN3/FD3_VCU0_0x1F0/LVBattVoltSta ==
  LVBattVoltSta : Inport
  Data Type Conversion : DataTypeConversion  OutDataTypeStr=uint8  RndMeth=Round
  CAN3_LVBattVoltSta : Outport
  wires:
  Data Type Conversion/1 -> CAN3_LVBattVoltSta/1
  LVBattVoltSta/1 -> Data Type Conversion/1

== system halout/HAL_OUT/CAN3/FD3_VCU0_0x1F0/LVChrgHoldTAct ==
  LVChrgHoldTAct : Inport
  Data Type Conversion : DataTypeConversion  OutDataTypeStr=uint16  RndMeth=Round
  CAN3_LVChrgHoldTAct : Outport
  wires:
  Data Type Conversion/1 -> CAN3_LVChrgHoldTAct/1
  LVChrgHoldTAct/1 -> Data Type Conversion/1

== system halout/HAL_OUT/CAN3/FD3_VCU0_0x1F0/LVSilentChrgLv ==
  LVSilentChrgLv : Inport
  Data Type Conversion : DataTypeConversion  OutDataTypeStr=uint8  RndMeth=Round
  CAN3_LVSilentChrgLv : Outport
  wires:
  Data Type Conversion/1 -> CAN3_LVSilentChrgLv/1
  LVSilentChrgLv/1 -> Data Type Conversion/1

== system halout/HAL_OUT/CAN3/FD3_VCU0_0x1F0/LVSilentChrgReq ==
  LVSilentChrgReq : Inport
  Data Type Conversion : DataTypeConversion  OutDataTypeStr=uint8  RndMeth=Round
  CAN3_LVSilentChrgReq : Outport
  wires:
  Data Type Conversion/1 -> CAN3_LVSilentChrgReq/1
  LVSilentChrgReq/1 -> Data Type Conversion/1

== system halout/HAL_OUT/CAN3/FD3_VCU0_0x1F0/LVSilentChrgSta ==
  LVSilentChrgSta : Inport
  Data Type Conversion : DataTypeConversion  OutDataTypeStr=uint8  RndMeth=Round
  CAN3_LVSilentChrgSta : Outport
  wires:
  Data Type Conversion/1 -> CAN3_LVSilentChrgSta/1
  LVSilentChrgSta/1 -> Data Type Conversion/1

== system halout/HAL_OUT/CAN3/FD3_VCU0_0x1F0/MCUActDisFail ==
  MCUActDisFail : Inport
  Data Type Conversion : DataTypeConversion  OutDataTypeStr=uint8  RndMeth=Round
  CAN3_MCUActDisFail : Outport
  wires:
  Data Type Conversion/1 -> CAN3_MCUActDisFail/1
  MCUActDisFail/1 -> Data Type Conversion/1

== system halout/HAL_OUT/CAN3/FD3_VCU0_0x1F0/PMMAllowECUSleep ==
  PMMAllowECUSleep : Inport
  Data Type Conversion : DataTypeConversion  OutDataTypeStr=uint8  RndMeth=Round
  CAN3_PMMAllowECUSleep : Outport
  wires:
  Data Type Conversion/1 -> CAN3_PMMAllowECUSleep/1
  PMMAllowECUSleep/1 -> Data Type Conversion/1

== system halout/HAL_OUT/CAN3/FD3_VCU0_0x1F0/PmicBootReason ==
  PmicBootReason : Inport
  Data Type Conversion : DataTypeConversion  OutDataTypeStr=uint8  RndMeth=Round
  CAN3_PmicBootReason : Outport
  wires:
  Data Type Conversion/1 -> CAN3_PmicBootReason/1
  PmicBootReason/1 -> Data Type Conversion/1

== system halout/HAL_OUT/CAN3/FD3_VCU0_0x1F0/PowerDownFault ==
  PowerDownFault : Inport
  Data Type Conversion : DataTypeConversion  OutDataTypeStr=uint8  RndMeth=Round
  CAN3_PowerDownFault : Outport
  wires:
  Data Type Conversion/1 -> CAN3_PowerDownFault/1
  PowerDownFault/1 -> Data Type Conversion/1

== system halout/HAL_OUT/CAN3/FD3_VCU0_0x1F0/PowerDownState ==
  PowerDownState : Inport
  Data Type Conversion : DataTypeConversion  OutDataTypeStr=uint8  RndMeth=Round
  CAN3_PowerDownState : Outport
  wires:
  Data Type Conversion/1 -> CAN3_PowerDownState/1
  PowerDownState/1 -> Data Type Conversion/1

== system halout/HAL_OUT/CAN3/FD3_VCU0_0x1F0/PowerUpFault ==
  PowerUpFault : Inport
  Data Type Conversion : DataTypeConversion  OutDataTypeStr=uint8  RndMeth=Round
  CAN3_PowerUpFault : Outport
  wires:
  Data Type Conversion/1 -> CAN3_PowerUpFault/1
  PowerUpFault/1 -> Data Type Conversion/1

== system halout/HAL_OUT/CAN3/FD3_VCU0_0x1F0/PowerUpState ==
  PowerUpState : Inport
  Data Type Conversion : DataTypeConversion  OutDataTypeStr=uint8  RndMeth=Round
  CAN3_PowerUpState : Outport
  wires:
  Data Type Conversion/1 -> CAN3_PowerUpState/1
  PowerUpState/1 -> Data Type Conversion/1

== system halout/HAL_OUT/CAN3/FD3_VCU0_0x1F0/PwrDownReq ==
  PwrDownReq : Inport
  Data Type Conversion : DataTypeConversion  OutDataTypeStr=uint8  RndMeth=Round
  CAN3_PwrDownReq : Outport
  wires:
  Data Type Conversion/1 -> CAN3_PwrDownReq/1
  PwrDownReq/1 -> Data Type Conversion/1

== system halout/HAL_OUT/CAN3/FD3_VCU0_0x1F0/PwrStaConstraint ==
  PwrStaConstraint : Inport
  Data Type Conversion : DataTypeConversion  OutDataTypeStr=uint8  RndMeth=Round
  CAN3_PwrStaConstraint : Outport
  wires:
  Data Type Conversion/1 -> CAN3_PwrStaConstraint/1
  PwrStaConstraint/1 -> Data Type Conversion/1

== system halout/HAL_OUT/CAN3/FD3_VCU0_0x1F0/PwrStaONTOIVIPopReq ==
  PwrStaONTOIVIPopReq : Inport
  Data Type Conversion : DataTypeConversion  OutDataTypeStr=uint8  RndMeth=Round
  CAN3_PwrStaONTOIVIPopReq : Outport
  wires:
  Data Type Conversion/1 -> CAN3_PwrStaONTOIVIPopReq/1
  PwrStaONTOIVIPopReq/1 -> Data Type Conversion/1

== system halout/HAL_OUT/CAN3/FD3_VCU0_0x1F0/PwrStaONTOIVIPopT ==
  PwrStaONTOIVIPopT : Inport
  Data Type Conversion : DataTypeConversion  OutDataTypeStr=uint16  RndMeth=Round
  CAN3_PwrStaONTOIVIPopT : Outport
  wires:
  Data Type Conversion/1 -> CAN3_PwrStaONTOIVIPopT/1
  PwrStaONTOIVIPopT/1 -> Data Type Conversion/1

== system halout/HAL_OUT/CAN3/FD3_VCU0_0x1F0/PwrStaSelect ==
  PwrStaSelect : Inport
  Data Type Conversion : DataTypeConversion  OutDataTypeStr=uint8  RndMeth=Round
  CAN3_PwrStaSelect : Outport
  wires:
  Data Type Conversion/1 -> CAN3_PwrStaSelect/1
  PwrStaSelect/1 -> Data Type Conversion/1

== system halout/HAL_OUT/CAN3/FD3_VCU0_0x1F0/PwrStaTOSta ==
  PwrStaTOSta : Inport
  Data Type Conversion : DataTypeConversion  OutDataTypeStr=uint8  RndMeth=Round
  CAN3_PwrStaTOSta : Outport
  wires:
  Data Type Conversion/1 -> CAN3_PwrStaTOSta/1
  PwrStaTOSta/1 -> Data Type Conversion/1

== system halout/HAL_OUT/CAN3/FD3_VCU0_0x1F0/PwrUpReq ==
  PwrUpReq : Inport
  Data Type Conversion : DataTypeConversion  OutDataTypeStr=uint8  RndMeth=Round
  CAN3_PwrUpReq : Outport
  wires:
  Data Type Conversion/1 -> CAN3_PwrUpReq/1
  PwrUpReq/1 -> Data Type Conversion/1

== system halout/HAL_OUT/CAN3/FD3_VCU0_0x1F0/RrTqSource ==
  RrTqSource : Inport
  Data Type Conversion : DataTypeConversion  OutDataTypeStr=uint8  RndMeth=Round
  CAN3_Rr_TqSource : Outport
  wires:
  Data Type Conversion/1 -> CAN3_Rr_TqSource/1
  RrTqSource/1 -> Data Type Conversion/1

== system halout/HAL_OUT/CAN3/FD3_VCU0_0x1F0/SchedChgTOSta ==
  SchedChgTOSta : Inport
  Data Type Conversion : DataTypeConversion  OutDataTypeStr=uint8  RndMeth=Round
  CAN3_SchedChgTOSta : Outport
  wires:
  Data Type Conversion/1 -> CAN3_SchedChgTOSta/1
  SchedChgTOSta/1 -> Data Type Conversion/1

== system halout/HAL_OUT/CAN3/FD3_VCU0_0x1F0/SilentChkAllowSleep ==
  SilentChkAllowSleep : Inport
  Data Type Conversion : DataTypeConversion  OutDataTypeStr=uint8  RndMeth=Round
  CAN3_SilentChkAllowSleep : Outport
  wires:
  Data Type Conversion/1 -> CAN3_SilentChkAllowSleep/1
  SilentChkAllowSleep/1 -> Data Type Conversion/1

== system halout/HAL_OUT/CAN3/FD3_VCU0_0x1F0/Subsystem ==
  s8_AcoreReadyToSleep : Inport
  VOUTP_CurrentNmState_enum : Inport  Port=2
  VOUTP_OTAPwrReqOFFChkSta_enum : Inport  Port=3
  VOUTP_OTAPwrReqStdChkSta_enum : Inport  Port=4
  Bitwise AND : simulink/Logic and Bit Operations/Bitwise Operator  logicop=AND  UseBitMask=on  BitMask=bin2dec('11111111')  BitMaskRealWorld=Stored Integer
  Bitwise AND1 : simulink/Logic and Bit Operations/Bitwise Operator  logicop=AND  UseBitMask=on  BitMask=bin2dec('11111111')  BitMaskRealWorld=Stored Integer
  Bitwise AND2 : simulink/Logic and Bit Operations/Bitwise Operator  logicop=AND  UseBitMask=on  BitMask=bin2dec('11111111')  BitMaskRealWorld=Stored Integer
  Bitwise OR2 : simulink/Logic and Bit Operations/Bitwise Operator  logicop=OR  UseBitMask=off  NumInputPorts=4  BitMask=bin2dec('00000000000000000000')  BitMaskRealWorld=Stored Integer
  Gain : Gain  Gain=50  OutDataTypeStr=single
  Saturation : Saturate  UpperLimit=1  LowerLimit=0  OutDataTypeStr=uint8
  Saturation1 : Saturate  UpperLimit=7  LowerLimit=0  OutDataTypeStr=uint8
  Saturation2 : Saturate  UpperLimit=3  LowerLimit=0  OutDataTypeStr=uint8
  Saturation3 : Saturate  UpperLimit=3  LowerLimit=0  OutDataTypeStr=uint8
  Shift Arithmetic6 : ArithShift  BitShiftNumber=1  BitShiftDirection=Left
  Shift Arithmetic7 : ArithShift  BitShiftNumber=4  BitShiftDirection=Left
  Shift Arithmetic8 : ArithShift  BitShiftNumber=6  BitShiftDirection=Left
  VehHVPwrAvail4THCM : Outport
  wires:
  Bitwise AND2/1 -> Bitwise OR2/2
  Shift Arithmetic6/1 -> Bitwise AND2/1
  Bitwise AND1/1 -> Bitwise OR2/3
  Shift Arithmetic7/1 -> Bitwise AND1/1
  Bitwise AND/1 -> Bitwise OR2/4
  Shift Arithmetic8/1 -> Bitwise AND/1
  Saturation3/1 -> Shift Arithmetic8/1
  Saturation2/1 -> Shift Arithmetic7/1
  Saturation/1 -> Bitwise OR2/1
  Saturation1/1 -> Shift Arithmetic6/1
  Gain/1 -> VehHVPwrAvail4THCM/1
  Bitwise OR2/1 -> Gain/1
  VOUTP_OTAPwrReqStdChkSta_enum/1 -> Saturation3/1
  VOUTP_OTAPwrReqOFFChkSta_enum/1 -> Saturation2/1
  VOUTP_CurrentNmState_enum/1 -> Saturation1/1
  s8_AcoreReadyToSleep/1 -> Saturation/1

== system halout/HAL_OUT/CAN3/FD3_VCU0_0x1F0/SysAllowReadySta ==
  SysAllowReadySta : Inport
  Data Type Conversion : DataTypeConversion  OutDataTypeStr=uint8  RndMeth=Round
  CAN3_SysAllowReadySta : Outport
  wires:
  Data Type Conversion/1 -> CAN3_SysAllowReadySta/1
  SysAllowReadySta/1 -> Data Type Conversion/1

== system halout/HAL_OUT/CAN3/FD3_VCU0_0x1F0/SysPwrSta ==
  SysPwrSta : Inport
  Data Type Conversion : DataTypeConversion  OutDataTypeStr=uint8  RndMeth=Round
  CAN3_SysPwrSta : Outport
  wires:
  Data Type Conversion/1 -> CAN3_SysPwrSta/1
  SysPwrSta/1 -> Data Type Conversion/1

== system halout/HAL_OUT/CAN3/FD3_VCU0_0x1F0/TCountSta ==
  TCountSta : Inport
  Data Type Conversion : DataTypeConversion  OutDataTypeStr=uint8  RndMeth=Round
  CAN3_TCountSta : Outport
  wires:
  Data Type Conversion/1 -> CAN3_TCountSta/1
  TCountSta/1 -> Data Type Conversion/1

== system halout/HAL_OUT/CAN3/FD3_VCU0_0x1F0/TimerAllowSleep ==
  TimerAllowSleep : Inport
  Data Type Conversion : DataTypeConversion  OutDataTypeStr=uint8  RndMeth=Round
  CAN3_TimerAllowSleep : Outport
  wires:
  Data Type Conversion/1 -> CAN3_TimerAllowSleep/1
  TimerAllowSleep/1 -> Data Type Conversion/1

== system halout/HAL_OUT/CAN3/FD3_VCU0_0x1F0/VCUBrkSWSta ==
  VCUBrkSWSta : Inport
  Data Type Conversion : DataTypeConversion  OutDataTypeStr=uint8  RndMeth=Round
  CAN3_VCUBrkSWSta : Outport
  wires:
  Data Type Conversion/1 -> CAN3_VCUBrkSWSta/1
  VCUBrkSWSta/1 -> Data Type Conversion/1

== system halout/HAL_OUT/CAN3/FD3_VCU0_0x1F0/VCUFLDoorSta ==
  VCUFLDoorSta : Inport
  Data Type Conversion : DataTypeConversion  OutDataTypeStr=uint8  RndMeth=Round
  CAN3_VCUFLDoorSta : Outport
  wires:
  Data Type Conversion/1 -> CAN3_VCUFLDoorSta/1
  VCUFLDoorSta/1 -> Data Type Conversion/1

== system halout/HAL_OUT/CAN3/FD3_VCU0_0x1F0/VCUFRDoorSta ==
  VCUFRDoorSta : Inport
  Data Type Conversion : DataTypeConversion  OutDataTypeStr=uint8  RndMeth=Round
  CAN3_VCUFRDoorSta : Outport
  wires:
  Data Type Conversion/1 -> CAN3_VCUFRDoorSta/1
  VCUFRDoorSta/1 -> Data Type Conversion/1

== system halout/HAL_OUT/CAN3/FD3_VCU0_0x1F0/VCURLDoorSta ==
  VCURLDoorSta : Inport
  Data Type Conversion : DataTypeConversion  OutDataTypeStr=uint8  RndMeth=Round
  CAN3_VCURLDoorSta : Outport
  wires:
  Data Type Conversion/1 -> CAN3_VCURLDoorSta/1
  VCURLDoorSta/1 -> Data Type Conversion/1

== system halout/HAL_OUT/CAN3/FD3_VCU0_0x1F0/VCURRDoorSta ==
  VCURRDoorSta : Inport
  Data Type Conversion : DataTypeConversion  OutDataTypeStr=uint8  RndMeth=Round
  CAN3_VCURRDoorSta : Outport
  wires:
  Data Type Conversion/1 -> CAN3_VCURRDoorSta/1
  VCURRDoorSta/1 -> Data Type Conversion/1

== system halout/HAL_OUT/CAN3/FD3_VCU0_0x1F0/VehHVPwrAvail4THCM ==
  VehHVPwrAvail4THCM : Inport
  Data Type Conversion : DataTypeConversion  OutDataTypeStr=uint8  RndMeth=Round
  convert_out : FVT_lib/hal/convert_out  gain=50  offset=0
  CAN3_VehHVPwrAvail4THCM : Outport
  wires:
  Data Type Conversion/1 -> CAN3_VehHVPwrAvail4THCM/1
  convert_out/1 -> Data Type Conversion/1
  VehHVPwrAvail4THCM/1 -> convert_out/1

== system halout/HAL_OUT/CAN3/FD3_VCU0_0x1F0/WisrBootReason ==
  WisrBootReason : Inport
  Data Type Conversion : DataTypeConversion  OutDataTypeStr=uint32  RndMeth=Round
  CAN3_WisrBootReason : Outport
  wires:
  Data Type Conversion/1 -> CAN3_WisrBootReason/1
  WisrBootReason/1 -> Data Type Conversion/1

== system halout/HAL_OUT/CAN3/FD3_VCU1_0x115/ActiveDischReq ==
  ActiveDischReq : Inport
  Data Type Conversion : DataTypeConversion  OutDataTypeStr=uint8  RndMeth=Round
  CAN3_ActiveDischReq : Outport
  wires:
  Data Type Conversion/1 -> CAN3_ActiveDischReq/1
  ActiveDischReq/1 -> Data Type Conversion/1

== system halout/HAL_OUT/CAN3/FD3_VCU1_0x115/CSVCU1 ==
  CSVCU1 : Inport
  Data Type Conversion : DataTypeConversion  OutDataTypeStr=uint8  RndMeth=Round
  CAN3_CS_VCU1 : Outport
  wires:
  Data Type Conversion/1 -> CAN3_CS_VCU1/1
  CSVCU1/1 -> Data Type Conversion/1

== system halout/HAL_OUT/CAN3/FD3_VCU1_0x115/CoastDwModeStaChk ==
  CoastDwModeStaChk : Inport
  Data Type Conversion : DataTypeConversion  OutDataTypeStr=uint8  RndMeth=Round
  CAN3_CoastDwModeStaChk : Outport
  wires:
  Data Type Conversion/1 -> CAN3_CoastDwModeStaChk/1
  CoastDwModeStaChk/1 -> Data Type Conversion/1

== system halout/HAL_OUT/CAN3/FD3_VCU1_0x115/DCDCEnaReq ==
  DCDCEnaReq : Inport
  Data Type Conversion : DataTypeConversion  OutDataTypeStr=uint8  RndMeth=Round
  CAN3_DCDCEnaReq : Outport
  wires:
  Data Type Conversion/1 -> CAN3_DCDCEnaReq/1
  DCDCEnaReq/1 -> Data Type Conversion/1

== system halout/HAL_OUT/CAN3/FD3_VCU1_0x115/DCDCVoltSetpoint ==
  DCDCVoltSetpoint : Inport
  Data Type Conversion : DataTypeConversion  OutDataTypeStr=uint8  RndMeth=Round
  convert_out : FVT_lib/hal/convert_out  gain=0.0235  offset=12
  CAN3_DCDCVoltSetpoint : Outport
  wires:
  Data Type Conversion/1 -> CAN3_DCDCVoltSetpoint/1
  convert_out/1 -> Data Type Conversion/1
  DCDCVoltSetpoint/1 -> convert_out/1

== system halout/HAL_OUT/CAN3/FD3_VCU1_0x115/DemoModeStaChk ==
  DemoModeStaChk : Inport
  Data Type Conversion : DataTypeConversion  OutDataTypeStr=uint8  RndMeth=Round
  CAN3_DemoModeStaChk : Outport
  wires:
  Data Type Conversion/1 -> CAN3_DemoModeStaChk/1
  DemoModeStaChk/1 -> Data Type Conversion/1

== system halout/HAL_OUT/CAN3/FD3_VCU1_0x115/DrSeatSta ==
  DrSeatSta : Inport
  Data Type Conversion : DataTypeConversion  OutDataTypeStr=uint8  RndMeth=Round
  CAN3_Dr_SeatSta : Outport
  wires:
  Data Type Conversion/1 -> CAN3_Dr_SeatSta/1
  DrSeatSta/1 -> Data Type Conversion/1

== system halout/HAL_OUT/CAN3/FD3_VCU1_0x115/DynoModeStaChk ==
  DynoModeStaChk : Inport
  Data Type Conversion : DataTypeConversion  OutDataTypeStr=uint8  RndMeth=Round
  CAN3_DynoModeStaChk : Outport
  wires:
  Data Type Conversion/1 -> CAN3_DynoModeStaChk/1
  DynoModeStaChk/1 -> Data Type Conversion/1

== system halout/HAL_OUT/CAN3/FD3_VCU1_0x115/HVBatCnctReq ==
  HVBatCnctReq : Inport
  Data Type Conversion : DataTypeConversion  OutDataTypeStr=uint8  RndMeth=Round
  CAN3_HVBatCnctReq : Outport
  wires:
  Data Type Conversion/1 -> CAN3_HVBatCnctReq/1
  HVBatCnctReq/1 -> Data Type Conversion/1

== system halout/HAL_OUT/CAN3/FD3_VCU1_0x115/HVSysReadyToCharge ==
  HVSysReadyToCharge : Inport
  Data Type Conversion : DataTypeConversion  OutDataTypeStr=uint8  RndMeth=Round
  CAN3_HVSysReadyToCharge : Outport
  wires:
  Data Type Conversion/1 -> CAN3_HVSysReadyToCharge/1
  HVSysReadyToCharge/1 -> Data Type Conversion/1

== system halout/HAL_OUT/CAN3/FD3_VCU1_0x115/LVChrgFuncStaChk ==
  LVChrgFuncStaChk : Inport
  Data Type Conversion : DataTypeConversion  OutDataTypeStr=uint8  RndMeth=Round
  CAN3_LVChrgFuncStaChk : Outport
  wires:
  Data Type Conversion/1 -> CAN3_LVChrgFuncStaChk/1
  LVChrgFuncStaChk/1 -> Data Type Conversion/1

== system halout/HAL_OUT/CAN3/FD3_VCU1_0x115/MSACrlSta ==
  MSACrlSta : Inport
  Data Type Conversion : DataTypeConversion  OutDataTypeStr=uint8  RndMeth=Round
  CAN3_MSA_Crl_Sta : Outport
  wires:
  Data Type Conversion/1 -> CAN3_MSA_Crl_Sta/1
  MSACrlSta/1 -> Data Type Conversion/1

== system halout/HAL_OUT/CAN3/FD3_VCU1_0x115/PButtonSta ==
  PButtonSta : Inport
  Data Type Conversion : DataTypeConversion  OutDataTypeStr=uint8  RndMeth=Round
  CAN3_P_Button_Sta : Outport
  wires:
  Data Type Conversion/1 -> CAN3_P_Button_Sta/1
  PButtonSta/1 -> Data Type Conversion/1
